simulink model "E_Netzwerk_2015a"  (R2015a)
settings: Solver=ode45  SolverMode=SingleTasking  StartTime=0.0  StopTime=10.0  RelTol=1e-3
values from neighbouring files (symbols this model uses):
  C1_ref = 1e-6    (= 1e-06)    [Esys_Parameter.m]    (also in aufgabe_1.m)
  C2 = 1e-6    (= 1e-06)    [Esys_Parameter.m]    (also in aufgabe_1.m)
  K = 3    [Esys_Parameter.m]    (also in aufgabe_1.m)
  kC1 = 800e-9    (= 8e-07)    [Esys_Parameter.m]    (also in aufgabe_1.m)
  R_1 = 625    [Esys_Parameter.m]    (also in aufgabe_1.m = tf(1,[1 0]); aufgabe_8.m = tf([1], [1 0]); aufgabe_9.m = 2.85714285714)
  R_2 = 3500    [Esys_Parameter.m]    (also in aufgabe_1.m = tf([T_2 1],1) * R_1; aufgabe_8.m = tf([T_I 1],1) * R_1)
  te = .05    (= 0.05)    [Esys_Parameter.m]    (also in aufgabe_1.m = 1)
  ts = .1    (= 0.1)    [Esys_Parameter.m]    (also in aufgabe_1.m = 3)
  UC1_ref = -10    [Esys_Parameter.m]    (also in aufgabe_1.m)
  UC1R = -(K*R2*UeR - R1*UsR - 2*R2*UeR + K*R1*UsR + K*R2*UsR)/(R1 + 2*R2)    (= -10)    [aufgabe_1.m]
  UC2R = (R2*UeR + R1*UsR + R2*UsR)/(R1 + 2*R2)    (= 5)    [aufgabe_1.m]
  Ue = 7    [Esys_Parameter.m]    (also in aufgabe_1.m)
  UeR = 5    [Esys_Parameter.m]    (also in aufgabe_1.m)
  Us = 4    [Esys_Parameter.m]    (also in aufgabe_1.m = 1)
  Usinus = 1    [Esys_Parameter.m]    (also in aufgabe_1.m = 0.1)
  UsR = 5    [Esys_Parameter.m]    (also in aufgabe_1.m)
  we = 1000    [Esys_Parameter.m]    (also in aufgabe_1.m = 10)
undefined symbols (not defined in the file or in its folder): k
libraries: cstblocks x4, simulink x1
settings Model: CovSFcnEnable=off  Creator=sj  LastModifiedBy=cha
settings OptimizationCC: BlockReduction=off  BooleanDataType=off
settings DebuggingCC: SaveWithParameterizedLinksMsg=none  UnderspecifiedInitializationDetection=Classic  MergeDetectMultiDrivingBlocksExec=none  SignalResolutionControl=TryResolveAllWithWarning  StrictBusMsg=Warning
settings HardwareCC: TargetUnknown=on

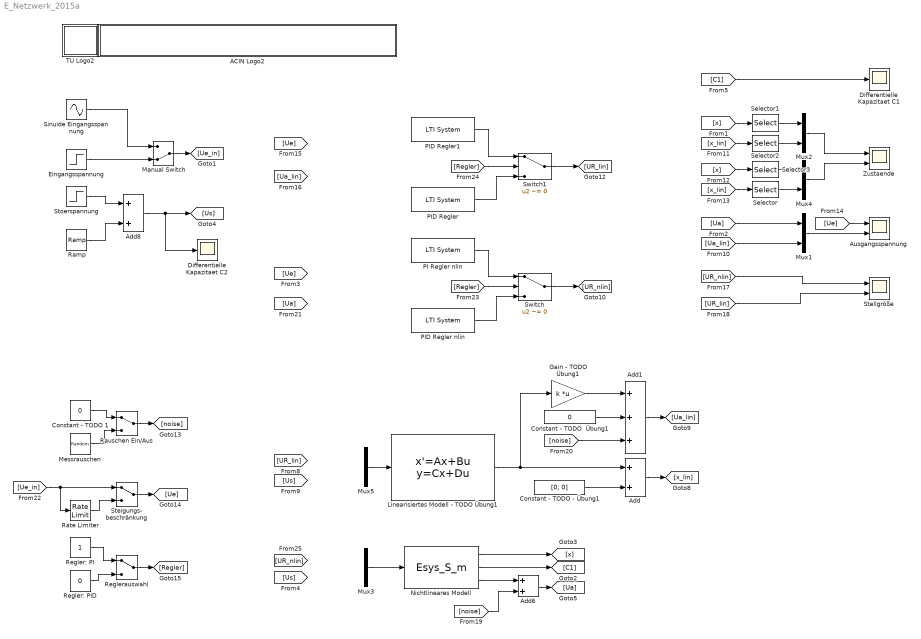
== system E_Netzwerk_2015a ==
  ACIN Logo2 : Subsystem
      mask init:
      | s = get_param(gcb,'UserData');
      mask Display:
      | image(s.logo,[0 0 439 45]);
      | %axis image
  Add : Sum
  Add1 : Sum  Inputs=+++
  Add6 : Sum
  Add8 : Sum
  Ausgangsspannung : Scope  NumInputPorts=2
      settings: TimeRange=auto  MaxDataPoints=5000  SaveToWorkspace=off  YMin=4.75~14.7252  YMax=7.25~17.47321  SampleTime=-1
  Constant - TODO  Übung1 : Constant  Value=0
  Constant - TODO - Übung1 : Constant  Value=[0; 0]
  Constant - TODO 1 : Constant  Value=0
  Differentielle Kapazitaet C1 : Scope
      settings: TimeRange=20  MaxDataPoints=5000  SaveToWorkspace=off  SaveName=ScopeData3  YMin=0.0000002  YMax=0.0000021  SampleTime=-1
  Differentielle Kapazitaet C2 : Scope
      settings: TimeRange=auto  MaxDataPoints=5000  SaveToWorkspace=off  YMin=3.8125  YMax=5.6875  SampleTime=-1
  Eingangsspannung : Step  Time=te  Before=UeR  After=Ue  SampleTime=0
  Gain - TODO Übung1 : Gain  Gain=k  Multiplication=Matrix(K*u)
  Linearisiertes Modell - TODO Übung1 : StateSpace  A=zeros(2)  B=zeros(2)  C=zeros(2)  D=zeros(2)  X0=[0;0]
  Manual Switch : ManualSwitch  CurrentSetting=0
  Messrauschen : UniformRandomNumber  Minimum=-5e-2  Maximum=5e-2  SampleTime=1e-3
  Mux{1..5} (5 alike) : Mux  Inputs=2
  Nichtlineares Modell : M-S-Function  FunctionName=Esys_S_m  Parameters=UC1R,UC2R,R_1,R_2,K,C1_ref,UC1_ref,kC1,C2
  PI Regler nlin : cstblocks/LTI System  sys=tf(1,[1 1])  IC=[]
  PID Regler : cstblocks/LTI System  sys=tf(1,[1 1])  IC=[]
  PID Regler nlin : cstblocks/LTI System  sys=tf(1,[1 1])  IC=[]
  PID Regler1 : cstblocks/LTI System  sys=tf(1,[1 1])  IC=[]
  Ramp : simulink/Sources/Ramp  slope=1  start=0  X0=0
  Rate Limiter : RateLimiter  RisingSlewLimit=100  FallingSlewLimit=-100  SampleTimeMode=inherited
  Rauschen Ein/Aus : ManualSwitch
  Regler: PI : Constant
  Regler: PID : Constant  Value=0
  Reglerauswahl : ManualSwitch
  Selector : Selector  InputPortWidth=2  IndexOptions=Index vector (dialog)  Indices=2  OutputSizes=1
  Selector1 : Selector  InputPortWidth=2  IndexOptions=Index vector (dialog)  Indices=1  OutputSizes=1
  Selector2 : Selector  InputPortWidth=2  IndexOptions=Index vector (dialog)  Indices=1  OutputSizes=1
  Selector3 : Selector  InputPortWidth=2  IndexOptions=Index vector (dialog)  Indices=2  OutputSizes=1
  Sinuide Eingangsspannung : Sin  Amplitude=Usinus  Bias=UeR  Frequency=we  SampleTime=0
  Steigungs- beschränkung : ManualSwitch
  Stellgröße : Scope  NumInputPorts=2
      settings: TimeRange=auto  MaxDataPoints=5000  SaveToWorkspace=off  SaveName=ScopeData  YMin=4.61004~-0.33747  YMax=8.15988~3.03725  SampleTime=-1
  Stoerspannung : Step  Time=ts  Before=UsR  After=Us  SampleTime=0
  Switch : Switch  Criteria=u2 ~= 0
  Switch1 : Switch  Criteria=u2 ~= 0
  TU Logo2 : Subsystem
      mask init:
      | s = get_param(gcb,'UserData');
      mask Display: image(s.logo,[0 0 45 45]);
  Zustaende : Scope  NumInputPorts=2
      settings: TimeRange=auto  MaxDataPoints=5000  SaveToWorkspace=off  SaveName=ScopeData2  YMin=-11.00753~4.90778  YMax=-8.681~5.82995  SampleTime=-1
  wires:
  Nichtlineares Modell/1 -> [x]
  Nichtlineares Modell/2 -> [C1]
  Eingangsspannung/1 -> Manual Switch/2
  Sinuide Eingangsspannung/1 -> Manual Switch/1
  Manual Switch/1 -> [Ue_in]
  [C1] -> Differentielle Kapazitaet C1/1
  Linearisiertes Modell - TODO Übung1/1 -> Gain - TODO Übung1/1, Add/1
  Mux5/1 -> Linearisiertes Modell - TODO Übung1/1
  Add/1 -> [x_lin]
  Constant - TODO - Übung1/1 -> Add/2
  Gain - TODO Übung1/1 -> Add1/1
  Add1/1 -> [Ua_lin]
  [Ua] -> Mux1/1
  [Ua_lin] -> Mux1/2
  Selector1/1 -> Mux2/1
  Selector2/1 -> Mux2/2
  [x] -> Selector1/1
  [x_lin] -> Selector2/1
  Selector3/1 -> Mux4/1
  Selector/1 -> Mux4/2
  [x] -> Selector3/1
  [x_lin] -> Selector/1
  Mux2/1 -> Zustaende/1
  Mux4/1 -> Zustaende/2
  [Ue] -> Ausgangsspannung/1
  Mux1/1 -> Ausgangsspannung/2
  [UR_nlin] -> Stellgröße/1
  [UR_lin] -> Stellgröße/2
  ? -> PI Regler nlin/1, PID Regler nlin/1
  Mux3/1 -> Nichtlineares Modell/1
  Messrauschen/1 -> Rauschen Ein/Aus/2
  Constant - TODO 1/1 -> Rauschen Ein/Aus/1
  Rauschen Ein/Aus/1 -> [noise]
  Add6/1 -> [Ua]
  Nichtlineares Modell/3 -> Add6/1
  [noise] -> Add6/2
  [noise] -> Add1/3
  Steigungs- beschränkung/1 -> [Ue]
  [Ue_in] -> Rate Limiter/1, Steigungs- beschränkung/1
  Rate Limiter/1 -> Steigungs- beschränkung/2
  PI Regler nlin/1 -> Switch/1
  [Regler] -> Switch/2
  Regler: PID/1 -> Reglerauswahl/2
  Regler: PI/1 -> Reglerauswahl/1
  Reglerauswahl/1 -> [Regler]
  PID Regler nlin/1 -> Switch/3
  PID Regler1/1 -> Switch1/1
  [Regler] -> Switch1/2
  PID Regler/1 -> Switch1/3
  Switch1/1 -> [UR_lin]
  Stoerspannung/1 -> Add8/1
  Ramp/1 -> Add8/2
  Add8/1 -> Differentielle Kapazitaet C2/1, [Us]
  Switch/1 -> [UR_nlin]
  ? -> PID Regler1/1, PID Regler/1
  Constant - TODO  Übung1/1 -> Add1/2

== system E_Netzwerk_2015a/ACIN Logo2 ==

== system E_Netzwerk_2015a/TU Logo2 ==
